simulink model "model"  (R2016a)
settings: Solver=VariableStepAuto  StartTime=0.0  StopTime=50  RelTol=1e-3
settings Model: Creator=Lucas  LastModifiedBy=Lucas

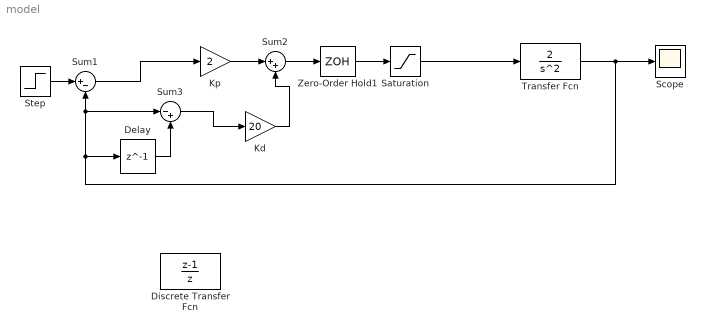
== system model ==
  Delay : Delay  DelayLength=1  InitialCondition=0  SampleTime=0.05
  Discrete Transfer Fcn : DiscreteTransferFcn  Numerator=[1 -1]  Denominator=[1 0]  SampleTime=0.05
  "Kd " : Gain  Gain=20
  "Kp " : Gain  Gain=2
  Saturation : Saturate  UpperLimit=0.1  LowerLimit=-0.1
  Scope : Scope
  Step : Step  After=0.05  SampleTime=0
  Sum1 : Sum  Inputs=|+-
  Sum2 : Sum  Inputs=|++
  Sum3 : Sum  Inputs=|-+
  Transfer Fcn : TransferFcn  Numerator=[2]  Denominator=[1 0 0]
  Zero-Order Hold1 : ZeroOrderHold  SampleTime=0.05
  wires:
  Transfer Fcn/1 -> Delay/1, Sum3/1, Sum1/2, Scope/1
  Step/1 -> Sum1/1
  Sum1/1 -> "Kp "/1
  "Kd "/1 -> Sum2/2
  "Kp "/1 -> Sum2/1
  Sum2/1 -> Zero-Order Hold1/1
  Zero-Order Hold1/1 -> Saturation/1
  Saturation/1 -> Transfer Fcn/1
  Delay/1 -> Sum3/2
  Sum3/1 -> "Kd "/1
